simulink model "Project26"  (R2023b)
settings: Solver=ode4  StartTime=0.0  StopTime=4*pi/n  FixedStep=0.1  RelTol=1e-3
values from neighbouring files (symbols this model uses):
  A = [A1; A2; A3; A4; A5; A6; A7; A8; A9; A10; A11; A12; A13; A14]    [Main.m]
  a = (509.4*1000+R_E+529.9*1000+R_E)/2    [Main.m]
  A_ssb = zeros(3,3,6)    [Main.m]
  e = 0.00149    [Main.m]
  epsilon = deg2rad(23.45)    [Main.m]
  F_e = 1358+600+150    (= 2108)    [Main.m]
  FOV = deg2rad(114)    [Main.m]
  G = 6.67*10^-11    (= 6.67e-11)    [Main.m]
  I = [Ix 0 0; 0 Iy 0; 0 0 Iz]    [Main.m]
  i = deg2rad(97.525)    [Main.m]
  I_inv = inv(I)    [Main.m]
  Ix = 0.13    [Main.m]
  Iy = 0.16    [Main.m]
  Iz = 0.18    [Main.m]
  j_B = [0.01, 0.05, 0.01]'    [Main.m]
  Mt = 5.97219e24    (= 5.97219e+24)    [Main.m]
  n = sqrt(G*Mt/a^3)    [Main.m]
  N_B = [n1; n2; n3; n4; n5; n6; n7; n8; n9; n10;n11;n12;n13;n14]    [Main.m]
  n_sun = 2*pi/T_earth    (= 1.99238499086e-07)    [Main.m]
  OM = deg2rad(6.934*180/12)    [Main.m]
  om = deg2rad(287.373)    [Main.m]
  q0 = [0 0 0 1]    [Main.m]
  r_CG = [0.02 0 0]    [Main.m]
  R_sun = astroConstants(2)*1e3    [Main.m]
  rF = [rF1; rF2; rF3; rF4; rF5; rF6; rF7; rF8; rF9; rF10;rF11;rF12;rF13;rF14]    [Main.m]
  theta0 = 0    [Main.m]
  Tsample = 0.1    [Main.m]
  w0 = [w_x0 w_y0 w_z0]    [Main.m]
  w_E = 7.291597763887421e-05    (= 7.29159776389e-05)    [Main.m]
  w_LN = [0 0 n]    [Main.m]
undefined symbols (not defined in the file or in its folder): actuators, control, DiscIntNeverNeededParam, environment, magnitude, sensors, settings
libraries: vrlib x6, matrix_library x5, simulink x2, aerolibutil x1
(part 1 of 2)
settings Model: Creator=aless  LastModifiedBy=aless

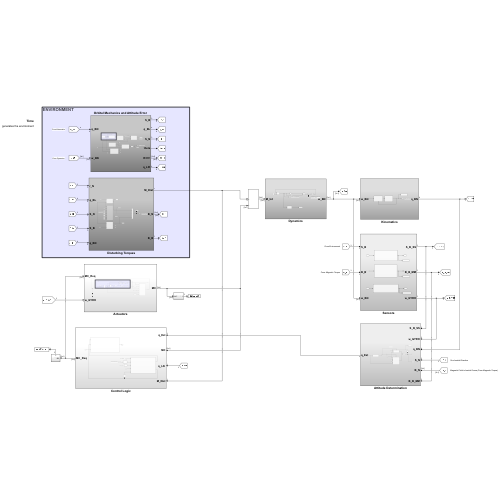
[thumbnail: Simulink's stored preview of the top-level diagram]
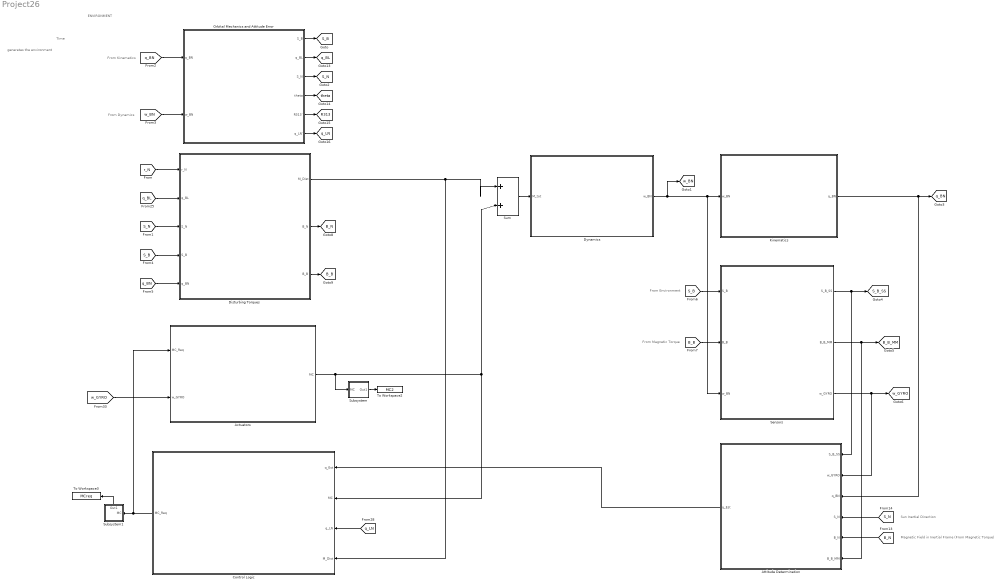
== system Project26 ==
  note: ENVIRONMENT
  note: generates the environment
  note: Time
  note: From Kinematics
  note: From Dynamics
  note: From Magnetic Torque
  note: From Environment
  note: Magnetic Field in Inertial Frame (From Magnetic Torque)
  note: Sun Inertial Direction
  Actuators : Subsystem
  Attitude Determination : Subsystem
  Control Logic : Subsystem
  Disturbing Torques : Subsystem
  Dynamics : Subsystem
  Kinematics : Subsystem
  "Orbital Mechanics and Attitude Error " : Subsystem
  Sensors : Subsystem
  Subsystem : Subsystem
  Subsystem1 : Subsystem
      settings: PortSchema="{\"entries\":[{\"content\":{\"sides\":[{\"content\":{},\"type\":\"ConnectorPlacement.EquallySpacedRectSide\",\"uuid\":\"79d52842-7462-4863-bae2-aaedde0a1e4a\"},{\"content\":{\"connectorIds\":[\"Out1\"],\"side\":\"RIGHT\"},\"type\":\"ConnectorPlacement.EquallySpacedRectSide\",\"uuid\":\"6db4fd27-b070-41dc-87e0-3dbfd9c74019\"},{\"content\":{\"side\":\"TOP\"},\"type\":\"ConnectorPlacement.EquallySpacedRectSide\",\"uuid\":\"0b737283-1eca-4b40-8e8f-9cc579166d68\"},{\"content\":{\"connectorIds\":[\"In1\"],\"side\":\"BOTTOM\"},\"type\":\"ConnectorPlacement.EquallySpacedRectSide\",\"uuid\":\"dd012077-7228-4314-a421-234f34c87179\"}]},\"type\":\"ConnectorPlacement.EquallySpacedConnector\",\"uuid\":\"e026e30a-a92e-42fe-b6eb-86c750f20789\"}],\"packageUris\":[\"http://schema.mathworks.com/mf0/Connector/R2020b\"],\"version\":\"1.0\"}"
  Sum : Sum  Inputs=|++
  To Workspace2 : ToWorkspace  VariableName=MC2  SampleTime=-1
  To Workspace3 : ToWorkspace  VariableName=MCreq  SampleTime=-1
  tag scope: B_B=global, B_B_MM=global, B_N=global, R313=global, S_B=global, S_B_SS=global, S_N=global, q_BL=global, q_BN=global, q_LN=global, theta=global, w_BN=global, w_GYRO=global
  wires:
  [w_BN] -> "Orbital Mechanics and Attitude Error "/2(w_BN)
  [q_BN] -> "Orbital Mechanics and Attitude Error "/1(q_BN)
  "Orbital Mechanics and Attitude Error "/1(S_B) -> [S_B]
  [S_N] -> Disturbing Torques/3(S_N)
  [r_N] -> Disturbing Torques/1(r_N)
  [S_B] -> Disturbing Torques/4(S_B)
  [q_BN] -> Disturbing Torques/5(q_BN)
  "Orbital Mechanics and Attitude Error "/3(S_N) -> [S_N]
  Kinematics/1(q_BN) -> Attitude Determination/3(q_BN), [q_BN]
  [S_B] -> Sensors/1(S_B)
  [B_B] -> Sensors/2(B_B)
  Sensors/1(S_B_SS) -> [S_B_SS], Attitude Determination/1(S_B_SS)
  Sensors/2(B_B_MM) -> [B_B_MM], Attitude Determination/6(B_B_MM)
  Sensors/3(w_GYRO) -> [w_GYRO], Attitude Determination/2(w_GYRO)
  Disturbing Torques/2(B_N) -> [B_N]
  Disturbing Torques/3(B_B) -> [B_B]
  Sum/1 -> Dynamics/1(M_tot)
  "Orbital Mechanics and Attitude Error "/2(q_BL) -> [q_BL]
  [q_BL] -> Disturbing Torques/2(q_BL)
  "Orbital Mechanics and Attitude Error "/4(theta) -> [theta]
  "Orbital Mechanics and Attitude Error "/5(R313') -> [R313]
  "Orbital Mechanics and Attitude Error "/6(q_LN') -> [q_LN]
  [w_GYRO] -> Actuators/1(w_GYRO)
  Actuators/1(MC) -> Sum/2, Control Logic/2(MC), Subsystem/1(MC)
  Subsystem/1(Out1) -> To Workspace2/1
  Subsystem1/1(Out1) -> To Workspace3/1
  Disturbing Torques/1(M_Dist) -> Control Logic/4(M_Dist), Sum/1
  Dynamics/1(w_BN) -> [w_BN], Sensors/3(w_BN), Kinematics/1(w_BN)
  [B_N] -> Attitude Determination/5(B_N)
  [S_N] -> Attitude Determination/4(S_N)
  Attitude Determination/1(q_Est) -> Control Logic/1(q_Est)
  [q_LN] -> Control Logic/3("q_LN ")
  Control Logic/1(MC_Req) -> Subsystem1/1(MC), Actuators/2(MC_Req)

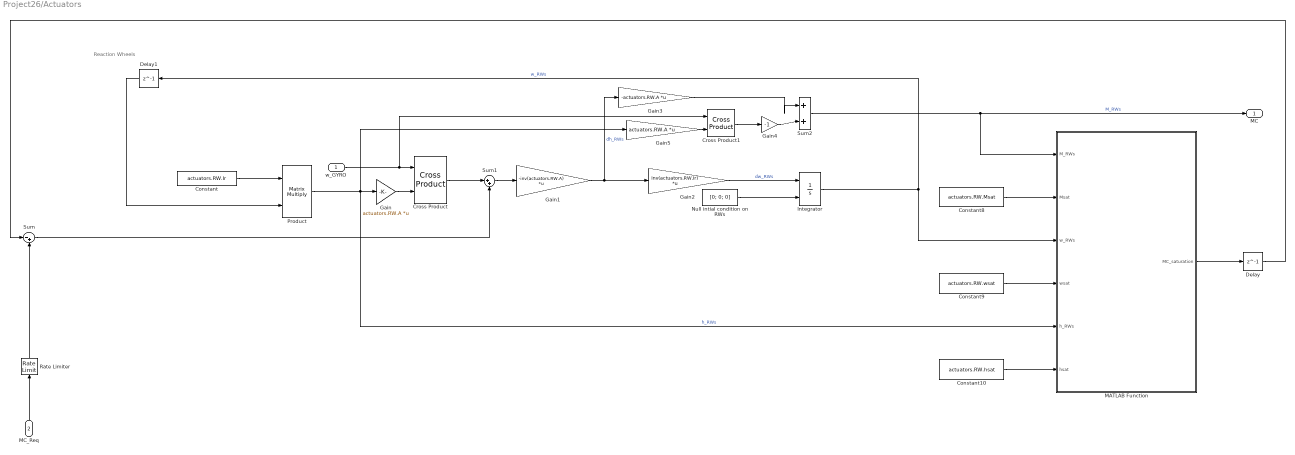
== system Project26/Actuators ==
  note: Reaction Wheels
  w_GYRO : Inport
  MC_Req : Inport  Port=2
  Constant : Constant  Value=actuators.RW.Ir
  Constant10 : Constant  Value=actuators.RW.hsat
  Constant8 : Constant  Value=actuators.RW.Msat
  Constant9 : Constant  Value=actuators.RW.wsat
  Cross Product : matrix_library/Cross Product
  Cross Product1 : matrix_library/Cross Product
  Delay : Delay  DelayLength=1
  Delay1 : Delay  DelayLength=1  InitialCondition=0
  Gain : Gain  Gain=actuators.RW.A  Multiplication=Matrix(K*u)
  Gain1 : Gain  Gain=-inv(actuators.RW.A)  Multiplication=Matrix(K*u)
  Gain2 : Gain  Gain=inv(actuators.RW.Ir)  Multiplication=Matrix(K*u)
  Gain3 : Gain  Gain=-actuators.RW.A  Multiplication=Matrix(K*u)
  Gain4 : Gain  Gain=-1
  Gain5 : Gain  Gain=actuators.RW.A  Multiplication=Matrix(K*u)
  Integrator : Integrator  InitialConditionSource=external
  MATLAB Function : MATLAB Function  TreatAsAtomicUnit=on
  Null intial condition on RWs : Constant  Value=[0; 0; 0]
  Product : Product  Multiplication=Matrix(*)
  Rate Limiter : RateLimiter
  Sum : Sum  Inputs=|-+
  Sum1 : Sum  Inputs=|++
  Sum2 : Sum  Inputs=|++
  MC : Outport
  wires:
  Sum/1 -> Sum1/2
  Sum2/1 -> MC/1, MATLAB Function/1(M_RWs)  "M_RWs"
  Gain2/1 -> Integrator/1  "dw_RWs"
  Gain3/1 -> Sum2/1
  Gain/1 -> Cross Product/2
  Delay1/1 -> Product/2
  w_GYRO/1 -> Cross Product1/1, Cross Product/1
  Gain1/1 -> Gain2/1, Gain3/1  "dh_RWs"
  Constant/1 -> Product/1
  Constant10/1 -> MATLAB Function/6(hsat)
  Delay/1 -> Sum/1
  MATLAB Function/1(MC_saturation) -> Delay/1
  Integrator/1 -> MATLAB Function/3(w_RWs), Delay1/1  "w_RWs"
  Product/1 -> MATLAB Function/5(h_RWs), Gain/1, Gain5/1  "h_RWs"
  Sum1/1 -> Gain1/1
  Gain5/1 -> Cross Product1/2
  Constant8/1 -> MATLAB Function/2(Msat)
  Constant9/1 -> MATLAB Function/4(wsat)
  Cross Product1/1 -> Gain4/1
  Cross Product/1 -> Sum1/1
  Gain4/1 -> Sum2/2
  Null intial condition on RWs/1 -> Integrator/2
  MC_Req/1 -> Rate Limiter/1
  Rate Limiter/1 -> Sum/2

== system Project26/Attitude Determination ==
  note: YES (isNaN = true)
  S_B_SS : Inport
  w_GYRO : Inport  Port=2
  q_BN : Inport  Port=3
  S_N : Inport  Port=4
  B_N : Inport  Port=5
  B_B_MM : Inport  Port=6
  Delay : Delay  DelayLength=1
  Enabled Subsystem : Subsystem  TreatAsAtomicUnit=on
  Enabled Subsystem1 : Subsystem  TreatAsAtomicUnit=on
  Merge1 : Merge
  NOT (Change of condition) : Logic  Operator=NOT  IconShape=distinctive  AllPortsSameDT=off  OutDataTypeStr=boolean
  Out of FOV check : Subsystem
  To Workspace : ToWorkspace  VariableName=delay  SaveFormat=Timeseries  SampleTime=-1
  To Workspace9 : ToWorkspace  VariableName=q_Est  SampleTime=-1
  q_Est : Outport
  wires:
  S_B_SS/1 -> Enabled Subsystem1/5(S_B_SS), Out of FOV check/1(S_B_SS)
  Out of FOV check/1(Out1) -> NOT (Change of condition)/1, Enabled Subsystem/Enable
  w_GYRO/1 -> Enabled Subsystem/1(w_GYRO)
  q_BN/1 -> Enabled Subsystem1/1(q_BN), Enabled Subsystem/3(q_BN)
  Enabled Subsystem/1(q_est) -> Merge1/1
  Merge1/1 -> To Workspace9/1, q_Est/1, Delay/1
  Delay/1 -> To Workspace/1, Enabled Subsystem/2(q_0)
  Enabled Subsystem1/1(q_est) -> Merge1/2
  NOT (Change of condition)/1 -> Enabled Subsystem1/Enable
  S_N/1 -> Enabled Subsystem1/2(S_N)
  B_N/1 -> Enabled Subsystem1/3(B_N)
  B_B_MM/1 -> Enabled Subsystem1/4(B_B_MM)

== system Project26/Control Logic ==
  note: From Actuators
  note: From Attitude Determination
  note: From Gyroscopes
  q_Est : Inport
  MC : Inport  Port=2
  "q_LN " : Inport  Port=3
  M_Dist : Inport  Port=4
  Control Block : Subsystem
  Delay : Delay  DelayLength=1
  Normalize Vector2 : vrlib/Utilities/Normalize Vector  maxzero=0
  State Observer : Subsystem
  MC_Req : Outport
  wires:
  q_Est/1 -> Normalize Vector2/1
  [w_GYRO] -> State Observer/3(w_GYRO)
  Delay/1 -> State Observer/5(q_obs_delay)
  Normalize Vector2/1 -> State Observer/2(q_raw)
  Control Block/1(MC_Req) -> MC_Req/1
  State Observer/2(q_obs) -> Control Block/2(q_obs), Delay/1
  State Observer/1(w_obs) -> Control Block/1(w_obs)
  MC/1 -> State Observer/1(MC_est)
  "q_LN "/1 -> Control Block/3("q_LN ")
  M_Dist/1 -> State Observer/4(MD)

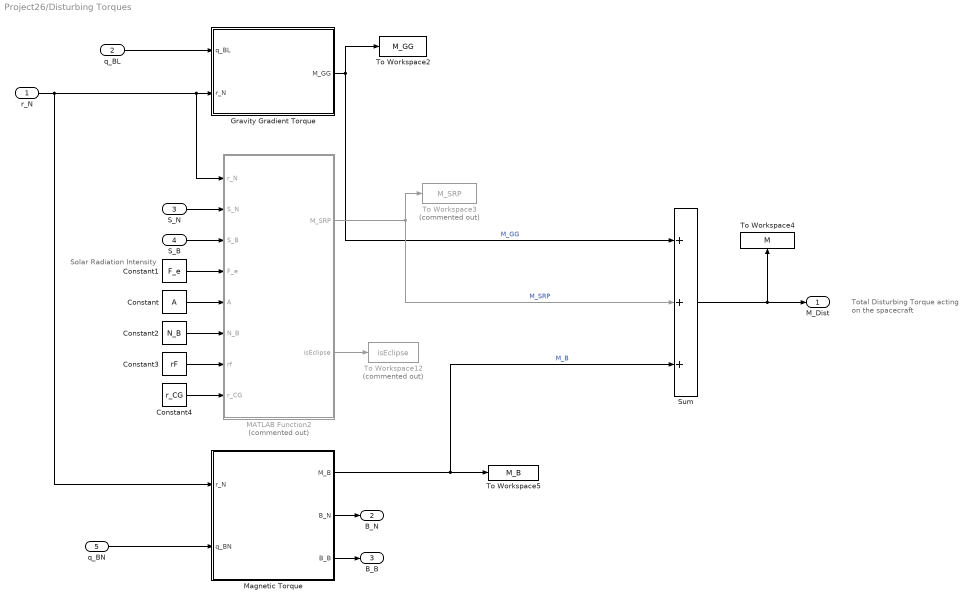
== system Project26/Disturbing Torques ==
  note: Total Disturbing Torque
      | acting on the spacecraft
  note: Solar Radiation Intensity
  r_N : Inport
  q_BL : Inport  Port=2
  S_N : Inport  Port=3
  S_B : Inport  Port=4
  q_BN : Inport  Port=5
  Constant : Constant  Value=A
  Constant1 : Constant  Value=F_e
  Constant2 : Constant  Value=N_B
  Constant3 : Constant  Value=rF
  Constant4 : Constant  Value=r_CG
  Gravity Gradient Torque : Subsystem
  MATLAB Function2 : MATLAB Function  Commented=on  TreatAsAtomicUnit=on
  Magnetic Torque : Subsystem
  Sum : Sum  Inputs=+++
  To Workspace12 : ToWorkspace  Commented=on  VariableName=isEclipse  SampleTime=-1
  To Workspace2 : ToWorkspace  VariableName=M_GG  SampleTime=-1
  To Workspace3 : ToWorkspace  Commented=on  VariableName=M_SRP  SampleTime=-1
  To Workspace4 : ToWorkspace  VariableName=M  SampleTime=-1
  To Workspace5 : ToWorkspace  VariableName=M_B  SampleTime=-1
  M_Dist : Outport
  B_N : Outport  Port=2
  B_B : Outport  Port=3
  wires:
  Constant1/1 -> MATLAB Function2/4(F_e)
  q_BL/1 -> Gravity Gradient Torque/1(q_BL)
  r_N/1 -> MATLAB Function2/1(r_N), Gravity Gradient Torque/2(r_N), Magnetic Torque/1(r_N)
  MATLAB Function2/2(isEclipse) -> To Workspace12/1
  q_BN/1 -> Magnetic Torque/2(q_BN)
  Sum/1 -> M_Dist/1, To Workspace4/1
  Gravity Gradient Torque/1(M_GG) -> To Workspace2/1, Sum/1  "M_GG"
  Magnetic Torque/1(M_B) -> Sum/3, To Workspace5/1  "M_B"
  S_N/1 -> MATLAB Function2/2(S_N)
  S_B/1 -> MATLAB Function2/3(S_B)
  Magnetic Torque/2(B_N) -> B_N/1
  Magnetic Torque/3(B_B) -> B_B/1
  Constant/1 -> MATLAB Function2/5(A)
  Constant2/1 -> MATLAB Function2/6(N_B)
  MATLAB Function2/1(M_SRP) -> To Workspace3/1, Sum/2  "M_SRP"
  Constant3/1 -> MATLAB Function2/7(rf)
  Constant4/1 -> MATLAB Function2/8(r_CG)

== system Project26/Dynamics ==
  note: Total Disturbing Torque+Control
      | acting on the spacecraft
  note: Angular velocity ( Body Frame )
  note: w
  M_tot : Inport
  Cross Product : vrlib/Utilities/Cross Product
  Gain : Gain  Gain=I  Multiplication=Matrix(K*u)
  Gain1 : Gain  Gain=I_inv  Multiplication=Matrix(K*u)
  Initial Condition : Constant  Value=w0
  Integrator : Integrator  InitialConditionSource=external
  Subsystem : Subsystem
  Sum : Sum  Inputs=|++
  To Workspace1 : ToWorkspace  VariableName=omega  SampleTime=-1
  w_BN : Outport
  wires:
  M_tot/1 -> Sum/2
  Gain1/1 -> Integrator/1
  Initial Condition/1 -> Integrator/2
  Sum/1 -> Gain1/1
  Gain/1 -> Cross Product/1  "I*w"
  Cross Product/1 -> Sum/1
  Integrator/1 -> Subsystem/1(MC), w_BN/1, Cross Product/2, Gain/1
  Subsystem/1(Out1) -> To Workspace1/1

== system Project26/Kinematics ==
  note: (Body Frame Quaternion)
  w_BN : Inport
  Quaternion Normalisation : Subsystem
  Quaternions : Subsystem
      settings: PortSchema="{\"entries\":[{\"content\":{\"sides\":[{\"content\":{\"connectorIds\":[\"In1\"]},\"type\":\"ConnectorPlacement.EquallySpacedRectSide\",\"uuid\":\"337480c7-b996-434a-97d1-93b75d8b293c\"},{\"content\":{\"connectorIds\":[\"Out1\"],\"side\":\"RIGHT\"},\"type\":\"ConnectorPlacement.EquallySpacedRectSide\",\"uuid\":\"41d32615-4344-48a4-ad5b-2dad4deabdda\"},{\"content\":{\"side\":\"TOP\"},\"type\":\"ConnectorPlacement.EquallySpacedRectSide\",\"uuid\":\"47835596-097d-48d1-90ae-77b48fddf76d\"},{\"content\":{\"connectorIds\":[\"In2\"],\"side\":\"BOTTOM\"},\"type\":\"ConnectorPlacement.EquallySpacedRectSide\",\"uuid\":\"9f38fa4d-c6c1-4321-9750-02b4f73c744f\"}]},\"type\":\"ConnectorPlacement.EquallySpacedConnector\",\"uuid\":\"8ea16f6d-57f4-43cd-ae9c-44a64026dd8f\"}],\"packageUris\":[\"http://schema.mathworks.com/mf0/Connector/R2020b\"],\"version\":\"1.0\"}"
  To Workspace : ToWorkspace  VariableName=q_BN  SampleTime=-1
  q_BN : Outport
  wires:
  w_BN/1 -> Quaternions/1(w)
  Quaternion Normalisation/1(q_BN) -> To Workspace/1, q_BN/1, Quaternions/2(q_BN)
  Quaternions/1(q(t)) -> Quaternion Normalisation/1(q(t))

== system Project26/Orbital Mechanics and Attitude Error  ==
  note: r_N = r ( Inertial Frame )
  note: Sun Direction ( Body Frame )
  note: r ( Body Frame )
  note: Two-Body Keplerian Dynamics
  q_BN : Inport
  w_BN : Inport  Port=2
  " Rotation from Inertial to Body Frame" : Subsystem
  Attitude Error : Subsystem
  Computation of r (vector) : Subsystem
  Normalize Vector : vrlib/Utilities/Normalize Vector  maxzero=0
  Rotation from Inertial to Body Frame : Subsystem
  Sun Inertial Direction : Subsystem
  Theta angle : Subsystem
  To Workspace : ToWorkspace  VariableName=r_B  SampleTime=-1
  To Workspace1 : ToWorkspace  VariableName=S_B  SampleTime=-1
  r (Magnitude) : Subsystem
  S_B : Outport
  q_BL : Outport  Port=2
  S_N : Outport  Port=3
  theta : Outport  Port=4
  R313' : Outport  Port=5
  q_LN' : Outport  Port=6
  wires:
  Theta angle/1(theta) -> Attitude Error/1(Theta), theta/1, Computation of r (vector)/2(theta), r (Magnitude)/1(theta)
  r (Magnitude)/1("r ") -> Computation of r (vector)/1(r)
  Computation of r (vector)/1(r_N) -> " Rotation from Inertial to Body Frame"/1(r_N)
  Sun Inertial Direction/1(S_N) -> Rotation from Inertial to Body Frame/1(S_N), S_N/1
  " Rotation from Inertial to Body Frame"/1(r_B) -> To Workspace/1
  Rotation from Inertial to Body Frame/1(S_B) -> Normalize Vector/1
  Normalize Vector/1 -> S_B/1, To Workspace1/1
  Attitude Error/1(q_BL) -> q_BL/1
  w_BN/1 -> Attitude Error/3(w_BN)
  q_BN/1 -> " Rotation from Inertial to Body Frame"/2(q_BN), Attitude Error/2(q_BN), Rotation from Inertial to Body Frame/2(q_BN)
  Computation of r (vector)/2(R313') -> R313'/1
  Attitude Error/2(q_LN') -> q_LN'/1

== system Project26/Sensors ==
  S_B : Inport
  B_B : Inport  Port=2
  w_BN : Inport  Port=3
  Gyroscopes : Subsystem
  Magnetometer : Subsystem
  Sun Sensor : Subsystem
      settings: PortSchema="{\"entries\":[{\"content\":{\"sides\":[{\"content\":{},\"type\":\"ConnectorPlacement.EquallySpacedRectSide\",\"uuid\":\"8c40b47c-c81f-4db9-9ecd-3bac70546829\"},{\"content\":{\"side\":\"RIGHT\"},\"type\":\"ConnectorPlacement.EquallySpacedRectSide\",\"uuid\":\"47b5da33-6a3e-4432-914f-62c5c8f09690\"},{\"content\":{\"connectorIds\":[\"In1\"],\"side\":\"TOP\"},\"type\":\"ConnectorPlacement.EquallySpacedRectSide\",\"uuid\":\"b24e362e-8249-41df-bcdf-30c7d216309c\"},{\"content\":{\"connectorIds\":[\"Out1\"],\"side\":\"BOTTOM\"},\"type\":\"ConnectorPlacement.EquallySpacedRectSide\",\"uuid\":\"ca1f88ba-b9cd-4169-975e-ff1bd0c05719\"}]},\"type\":\"ConnectorPlacement.EquallySpacedConnector\",\"uuid\":\"37a9beb8-71a0-43e5-b724-5b60e3432ba4\"}],\"packageUris\":[\"http://schema.mathworks.com/mf0/Connector/R2020b\"],\"version\":\"1.0\"}"
  To Workspace : ToWorkspace  VariableName=w_measured  SampleTime=-1
  To Workspace1 : ToWorkspace  VariableName=S_B_meas  SampleTime=-1
  To Workspace2 : ToWorkspace  VariableName=B_B_meas  SampleTime=-1
  S_B_SS : Outport
  B_B_MM : Outport  Port=2
  w_GYRO : Outport  Port=3
  wires:
  S_B/1 -> Sun Sensor/1(S_B)
  w_BN/1 -> Gyroscopes/1(w_BN)
  Sun Sensor/1(S_B_SS) -> S_B_SS/1, To Workspace1/1
  Magnetometer/1(B_B_MM) -> B_B_MM/1, To Workspace2/1
  Gyroscopes/1(w_GYRO) -> w_GYRO/1, To Workspace/1
  B_B/1 -> Magnetometer/1(B_B)

== system Project26/Subsystem ==
  MC : Inport
  Demux : Demux  Outputs=3
  Mux : Mux  Inputs=3
  Out1 : Outport
  wires:
  MC/1 -> Demux/1
  Demux/1 -> Mux/1
  Demux/2 -> Mux/2
  Demux/3 -> Mux/3
  Mux/1 -> Out1/1

== system Project26/Subsystem1 ==
  MC : Inport
  Demux : Demux  Outputs=3
  Mux : Mux  Inputs=3
  Out1 : Outport
  wires:
  MC/1 -> Demux/1
  Demux/1 -> Mux/1
  Demux/2 -> Mux/2
  Demux/3 -> Mux/3
  Mux/1 -> Out1/1

== system Project26/Attitude Determination/Enabled Subsystem ==
  note: Estimated
      | Quaternion
  w_GYRO : Inport
  q_0 : Inport  Port=2
  q_BN : Inport  Port=3
  Enable : EnablePort  StatesWhenEnabling=reset
  Kinematics : Subsystem
  Sign Determination : Subsystem
  To Workspace : ToWorkspace  VariableName=q_estG1  SampleTime=-1
  q_est : Outport
  wires:
  q_BN/1 -> Sign Determination/2(q_BN)
  w_GYRO/1 -> Kinematics/1(w)
  Kinematics/1(q_est) -> Sign Determination/1("q_est "), To Workspace/1
  q_0/1 -> Kinematics/2(q_0)
  Sign Determination/1(q_est) -> q_est/1

== system Project26/Attitude Determination/Enabled Subsystem1 ==
  note: S_B_Estim
  q_BN : Inport
  S_N : Inport  Port=2
  B_N : Inport  Port=3
  B_B_MM : Inport  Port=4
  S_B_SS : Inport  Port=5
  Enable : EnablePort
  Attitude determination : MATLAB Function  TreatAsAtomicUnit=on
  Constant : Constant  Value=sensors.mag.accuracy
  Constant2 : Constant  Value=sensors.SS.accuracy
  Normalize Vector1 : vrlib/Utilities/Normalize Vector  maxzero=0
  Sign determination : Subsystem
  q_est : Outport
  wires:
  Constant/1 -> Attitude determination/1(a_mag)
  q_BN/1 -> Sign determination/2(q_BN)
  Constant2/1 -> Attitude determination/2(a_sun)
  Normalize Vector1/1 -> Attitude determination/3(S_N)
  S_B_SS/1 -> Attitude determination/4(S_B_Estim)
  S_N/1 -> Normalize Vector1/1
  B_N/1 -> Attitude determination/5(B_N)
  B_B_MM/1 -> Attitude determination/6(B_B_Estim)
  Sign determination/1(q_0) -> q_est/1
  Attitude determination/1(q_est) -> Sign determination/1("q_est ")

== system Project26/Attitude Determination/Out of FOV check ==
  note: If at least one component is NaN, the Sun is not in the FOV
  S_B_SS : Inport
  Demux : Demux  Outputs=3
  IsNaN : RelationalOperator  Operator=isNaN  OutDataTypeStr=boolean  RndMeth=Simplest  InputSameDT=off
  Out1 : Outport
  wires:
  S_B_SS/1 -> Demux/1
  Demux/1 -> IsNaN/1
  IsNaN/1 -> Out1/1

== system Project26/Control Logic/Control Block ==
  note: Global Pointing Error
  note: Control Algorithms
  note: Mission Phase Decision
  w_obs : Inport
  q_obs : Inport  Port=2
  "q_LN " : Inport  Port=3
  Clock : Clock
  Constant : Constant  Value=control.detumbling.MaxTime
  Constant1 : Constant  Value=control.slewManeuvre.MaxTime
  Detumbling : Subsystem  TreatAsAtomicUnit=on
  If : If  NumInputs=3  IfExpression=u1<=u2  ElseIfExpressions=u2<u1<=u3
  Merge : Merge  Inputs=3
  Merge1 : Merge  Inputs=3
  Slew Maneuvre : Subsystem  TreatAsAtomicUnit=on
  To Workspace : ToWorkspace  VariableName=pointing_err  SampleTime=-1
  Trajectory Tracking : Subsystem  TreatAsAtomicUnit=on
  MC_Req : Outport
  wires:
  Constant1/1 -> If/3
  Constant/1 -> If/2
  Clock/1 -> If/1
  If/1 -> Detumbling/Action
  If/2 -> Slew Maneuvre/Action
  If/3 -> Trajectory Tracking/Action
  q_obs/1 -> Detumbling/2(q_obs), Trajectory Tracking/2(q_obs), Slew Maneuvre/2(q_obs)
  w_obs/1 -> Detumbling/1(w_obs), Trajectory Tracking/1(w_obs), Slew Maneuvre/1(w_obs)
  Trajectory Tracking/2(Pointing Error) -> Merge/1
  Slew Maneuvre/2(Pointing Error (SM)) -> Merge/2
  Detumbling/2(Pointing Error (DT)) -> Merge/3
  Merge/1 -> To Workspace/1
  Slew Maneuvre/1(MC) -> Merge1/2
  Trajectory Tracking/1(MC) -> Merge1/3
  Merge1/1 -> MC_Req/1  "MC_required"
  Detumbling/1(MC) -> Merge1/1
  "q_LN "/1 -> Detumbling/3(q_LN), Slew Maneuvre/3(q_LN), Trajectory Tracking/3(q_LN)

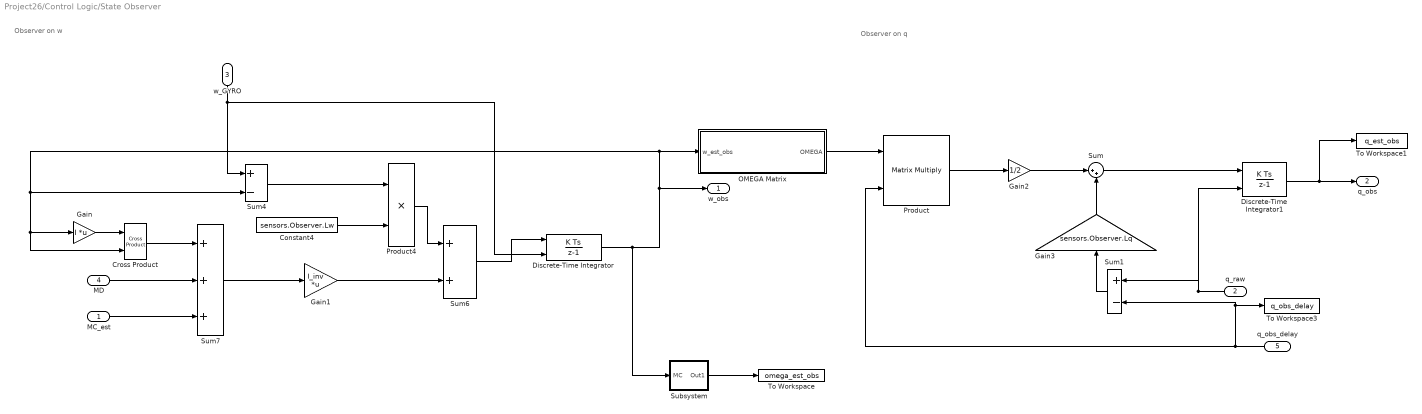
== system Project26/Control Logic/State Observer ==
  note: Observer on q
  note: Observer on w
  MC_est : Inport
  q_raw : Inport  Port=2
  w_GYRO : Inport  Port=3
  MD : Inport  Port=4
  q_obs_delay : Inport  Port=5
  Constant4 : Constant  Value=sensors.Observer.Lw
  Cross Product : vrlib/Utilities/Cross Product
  Discrete-Time Integrator : DiscreteIntegrator  InitialConditionSource=external  InitialCondition=sensors.Observer.w0  SampleTime=Tsample  ICPrevOutput=DiscIntNeverNeededParam  ICPrevScaledInput=DiscIntNeverNeededParam
  Discrete-Time Integrator1 : DiscreteIntegrator  InitialConditionSource=external  SampleTime=Tsample  ICPrevOutput=DiscIntNeverNeededParam  ICPrevScaledInput=DiscIntNeverNeededParam
  Gain : Gain  Gain=I  Multiplication=Matrix(K*u)
  Gain1 : Gain  Gain=I_inv  Multiplication=Matrix(K*u)
  Gain2 : Gain  Gain=1/2
  Gain3 : Gain  Gain=sensors.Observer.Lq
  OMEGA Matrix : Subsystem
  Product : Product  Multiplication=Matrix(*)
  Product4 : Product
  Subsystem : Subsystem
  Sum : Sum  Inputs=|++
  Sum1 : Sum  Inputs=|+-
  Sum4 : Sum  Inputs=+-
  Sum6 : Sum
  Sum7 : Sum  Inputs=+++
  To Workspace : ToWorkspace  VariableName=omega_est_obs  SampleTime=-1
  To Workspace1 : ToWorkspace  VariableName=q_est_obs  SampleTime=-1
  To Workspace3 : ToWorkspace  VariableName=q_obs_delay  SampleTime=-1
  w_obs : Outport
  q_obs : Outport  Port=2
  wires:
  Product4/1 -> Sum6/1
  Cross Product/1 -> Sum7/1
  Gain1/1 -> Sum6/2
  MC_est/1 -> Sum7/3
  Discrete-Time Integrator/1 -> Subsystem/1(MC), w_obs/1, Sum4/2, Gain/1, Cross Product/2, OMEGA Matrix/1(w_est_obs)
  Sum4/1 -> Product4/1
  Gain/1 -> Cross Product/1
  Constant4/1 -> Product4/2
  Sum7/1 -> Gain1/1
  w_GYRO/1 -> Discrete-Time Integrator/2, Sum4/1
  OMEGA Matrix/1(OMEGA) -> Product/1
  Product/1 -> Gain2/1
  Gain2/1 -> Sum/1
  Gain3/1 -> Sum/2
  Sum1/1 -> Gain3/1
  q_obs_delay/1 -> Sum1/2, To Workspace3/1, Product/2
  Sum/1 -> Discrete-Time Integrator1/1
  Sum6/1 -> Discrete-Time Integrator/1
  MD/1 -> Sum7/2
  Discrete-Time Integrator1/1 -> q_obs/1, To Workspace1/1
  q_raw/1 -> Discrete-Time Integrator1/2, Sum1/1
  Subsystem/1(Out1) -> To Workspace/1

== system Project26/Disturbing Torques/Gravity Gradient Torque ==
  note: Torque due to
      | Gravity Gradient
  note: c1c3
  note: c2c3
  note: c2c1
  note: c1,c2,c3
  q_BL : Inport
  r_N : Inport  Port=2
  Constant1 : Constant  Value=3
  Cubic Power : Math  Operator=pow
  Demux : Demux  Outputs=3
  Divide : Product  Inputs=*/
  Gain : Gain  Gain=(Iz-Iy)
  Gain1 : Gain  Gain=(Ix-Iz)
  Gain2 : Gain  Gain=(Iy-Ix)
  Gain7 : Gain  Gain=3*G*Mt
  Mux : Mux  Inputs=3
  Normalisation : Subsystem
  Product : Product
  Product1 : Product
  Product2 : Product
  Rotation of vector [1 0 0] : Subsystem
  Vector : Constant  Value=[1 0 0]'
  M_GG : Outport
  wires:
  Cubic Power/1 -> Divide/2
  Demux/1 -> Product1/1, Product2/2
  q_BL/1 -> Rotation of vector [1 0 0]/1(q_BL)
  Rotation of vector [1 0 0]/1(v_rot) -> Demux/1
  Normalisation/1(R) -> Cubic Power/1
  Divide/1 -> M_GG/1
  Vector/1 -> Rotation of vector [1 0 0]/2(Vector [1 0 0])  "vect"
  Product2/1 -> Gain2/1
  Demux/2 -> Product/1, Product2/1
  Mux/1 -> Gain7/1
  r_N/1 -> Normalisation/1(r_N)
  Gain7/1 -> Divide/1
  Demux/3 -> Product1/2, Product/2
  Constant1/1 -> Cubic Power/2
  Gain/1 -> Mux/1
  Gain1/1 -> Mux/2
  Gain2/1 -> Mux/3
  Product1/1 -> Gain1/1
  Product/1 -> Gain/1

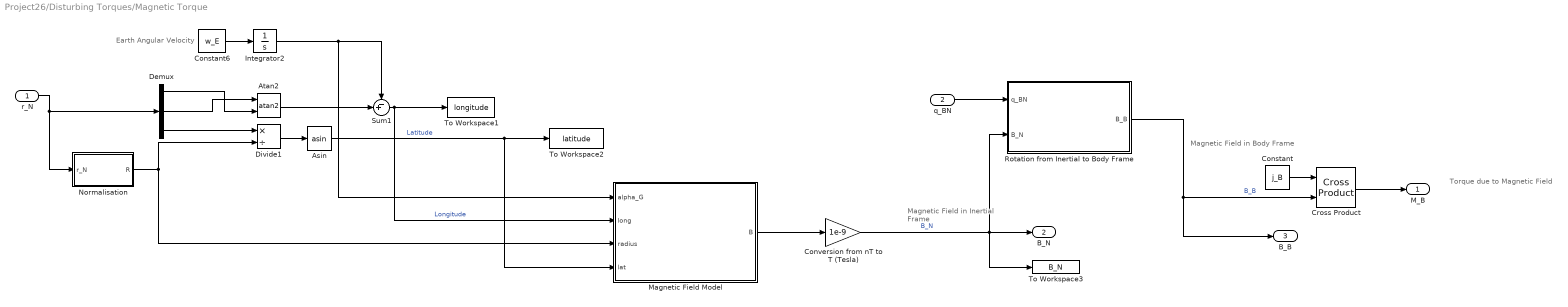
== system Project26/Disturbing Torques/Magnetic Torque ==
  note: Magnetic Field
      | in Body Frame
  note: Magnetic Field
      | in Inertial Frame
  note: Earth Angular Velocity
  note: Torque due to
      | Magnetic Field
  r_N : Inport
  q_BN : Inport  Port=2
  Asin : Trigonometry  Operator=asin
  Atan2 : Trigonometry  Operator=atan2
  Constant : Constant  Value=j_B
  Constant6 : Constant  Value=w_E
  Conversion from nT to T (Tesla) : Gain  Gain=1e-9
  Cross Product : matrix_library/Cross Product
  Demux : Demux  Outputs=3
  Divide1 : Product  Inputs=*/
  Integrator2 : Integrator
  Magnetic Field Model : MATLAB Function  TreatAsAtomicUnit=on
  Normalisation : Subsystem
  Rotation from Inertial to Body Frame : Subsystem
  Sum1 : Sum  Inputs=-+|
  To Workspace1 : ToWorkspace  VariableName=longitude  SampleTime=-1
  To Workspace2 : ToWorkspace  VariableName=latitude  SampleTime=-1
  To Workspace3 : ToWorkspace  VariableName=B_N  SampleTime=-1
  M_B : Outport
  B_N : Outport  Port=2
  B_B : Outport  Port=3
  wires:
  Demux/2 -> Atan2/1
  Demux/3 -> Divide1/1
  Atan2/1 -> Sum1/2
  Normalisation/1(R) -> Magnetic Field Model/3(radius), Divide1/2
  Demux/1 -> Atan2/2
  Divide1/1 -> Asin/1
  Asin/1 -> Magnetic Field Model/4(lat), To Workspace2/1  "Latitude"
  Constant6/1 -> Integrator2/1
  Sum1/1 -> To Workspace1/1, Magnetic Field Model/2(long)  "Longitude"
  r_N/1 -> Normalisation/1(r_N), Demux/1
  Integrator2/1 -> Sum1/1, Magnetic Field Model/1(alpha_G)
  Rotation from Inertial to Body Frame/1(B_B) -> B_B/1, Cross Product/2  "B_B"
  Constant/1 -> Cross Product/1
  Magnetic Field Model/1(B) -> Conversion from nT to T (Tesla)/1
  q_BN/1 -> Rotation from Inertial to Body Frame/1(q_BN)
  Cross Product/1 -> M_B/1
  Conversion from nT to T (Tesla)/1 -> B_N/1, Rotation from Inertial to Body Frame/2(B_N), To Workspace3/1  "B_N"

== system Project26/Dynamics/Subsystem ==
  MC : Inport
  Demux : Demux  Outputs=3
  Mux : Mux  Inputs=3
  Out1 : Outport
  wires:
  MC/1 -> Demux/1
  Demux/1 -> Mux/1
  Demux/2 -> Mux/2
  Demux/3 -> Mux/3
  Mux/1 -> Out1/1

== system Project26/Kinematics/Quaternion Normalisation ==
  q(t) : Inport
  Divide : Product  Inputs=*/
  Dot Product : DotProduct  OutDataTypeStr=Inherit: Inherit via internal rule
  Sqrt : Sqrt
  q_BN : Outport
  wires:
  Dot Product/1 -> Sqrt/1
  q(t)/1 -> Divide/1, Dot Product/1, Dot Product/2
  Sqrt/1 -> Divide/2
  Divide/1 -> q_BN/1

== system Project26/Kinematics/Quaternions ==
  note: Normalised
      | quaternion
  w : Inport
  q_BN : Inport  Port=2
  Gain : Gain  Gain=1/2
  Initial Condition : Constant  Value=q0
  Integrator : Integrator  InitialConditionSource=external
  Matrix Multiply : Product  Multiplication=Matrix(*)
  OMEGA Matrix : Subsystem
  q(t) : Outport
  wires:
  Integrator/1 -> q(t)/1
  Initial Condition/1 -> Integrator/2
  Matrix Multiply/1 -> Integrator/1
  Gain/1 -> Matrix Multiply/1
  w/1 -> OMEGA Matrix/1(w)
  OMEGA Matrix/1(OM Matrix) -> Gain/1
  q_BN/1 -> Matrix Multiply/2

== system Project26/Orbital Mechanics and Attitude Error / Rotation from Inertial to Body Frame ==
  note: Quaternion Rotation (Double Tensor Product)
  note: $\vec{r_B} = q_{BN}'\otimes [\vec{r_N};0]\otimes q_{BN}$
  r_N : Inport
  q_BN : Inport  Port=2
  Demux : Demux
  Mux : Mux  Inputs=3
  Quaternion multiplication 1 : Subsystem
  Quaternion multiplication 2 : Subsystem
  Transformation in Quaternion : Subsystem
  Transpose : Gain  Gain=[-1 -1 -1 1]
  r_B : Outport
  wires:
  r_N/1 -> Transformation in Quaternion/1(r_N)
  Mux/1 -> r_B/1
  Transpose/1 -> Quaternion multiplication 1/1(q_BN')
  q_BN/1 -> Quaternion multiplication 2/2(q_BN), Transpose/1
  Transformation in Quaternion/1(q(r_N)) -> Quaternion multiplication 1/2("q(r_N) ")
  Quaternion multiplication 2/1(q(r_B)) -> Demux/1
  Quaternion multiplication 1/1(q1) -> Quaternion multiplication 2/1(q1)
  Demux/1 -> Mux/1
  Demux/2 -> Mux/2
  Demux/3 -> Mux/3

== system Project26/Orbital Mechanics and Attitude Error /Attitude Error ==
  note: Angular Velocity Error
  note: Reference moving attitude
      | (Angular Velocity)
  note: Attitude Error
  note: Reference moving attitude
      | (Quaternion)
  Theta : Inport
  q_BN : Inport  Port=2
  w_BN : Inport  Port=3
  Computation of q_BL : Subsystem
  Constant2 : Constant  Value=w_LN
  Rotation of w_LN : Subsystem
  Sum : Sum  Inputs=|-+
  To Workspace3 : ToWorkspace  VariableName=w_BL  SampleTime=-1
  To Workspace4 : ToWorkspace  VariableName=q_BL  SampleTime=-1
  q_LN : Subsystem
  q_BL : Outport
  q_LN' : Outport  Port=2
  wires:
  Computation of q_BL/1(q_BL) -> Rotation of w_LN/1(q_BL), To Workspace4/1, q_BL/1
  Theta/1 -> q_LN/1(Theta)
  Sum/1 -> To Workspace3/1
  Rotation of w_LN/1(w_LN') -> Sum/1
  Constant2/1 -> Rotation of w_LN/2(w_LN)
  q_BN/1 -> q_LN/2(q_BN), Computation of q_BL/1(q_BN)
  q_LN/1(q_LN') -> Computation of q_BL/2(q_LN'), q_LN'/1
  w_BN/1 -> Sum/2

== system Project26/Orbital Mechanics and Attitude Error /Computation of r (vector) ==
  note: Perifocal Frame
  note: r (Perifocal Frame)
  r : Inport
  theta : Inport  Port=2
  Constant : Constant  Value=0
  Cos1 : Trigonometry  Operator=cos
  Mux1 : Mux  Inputs=3
  Product1 : Product  Multiplication=Matrix(*)
  Product2 : Product
  Rotation (R313') from Perifocal to ECI : Subsystem
  Sin1 : Trigonometry
  To Workspace1 : ToWorkspace  VariableName=r_N  SampleTime=-1
  r_N : Outport
  R313' : Outport  Port=2
  tag scope: r_N=global
  wires:
  Mux1/1 -> Product2/2
  Sin1/1 -> Mux1/2
  Constant/1 -> Mux1/3
  Rotation (R313') from Perifocal to ECI/1(R313) -> R313'/1, Product1/1
  Cos1/1 -> Mux1/1
  Product1/1 -> [r_N], r_N/1, To Workspace1/1
  theta/1 -> Sin1/1, Cos1/1
  r/1 -> Product2/1
  Product2/1 -> Product1/2

== system Project26/Orbital Mechanics and Attitude Error /Rotation from Inertial to Body Frame ==
  note: $\vec{S_B} = q_{BN}'\otimes [\vec{S_N};0]\otimes q_{BN}$
  note: Quaternion Rotation (Double Tensor Product)
  S_N : Inport
  q_BN : Inport  Port=2
  Demux : Demux
  Mux : Mux  Inputs=3
  Quaternion multiplication 1 : Subsystem
  Quaternion multiplication 2 : Subsystem
  Transformation in Quaternion : Subsystem
  Transpose : Gain  Gain=[-1 -1 -1 1]
  S_B : Outport
  wires:
  S_N/1 -> Transformation in Quaternion/1(S_N)
  Mux/1 -> S_B/1
  Transpose/1 -> Quaternion multiplication 1/1(q_BN')
  q_BN/1 -> Quaternion multiplication 2/2(q_BN), Transpose/1
  Transformation in Quaternion/1(q(S_N)) -> Quaternion multiplication 1/2(q(S_N))
  Quaternion multiplication 2/1(q(S_B)) -> Demux/1
  Quaternion multiplication 1/1(q1) -> Quaternion multiplication 2/1(q1)
  Demux/1 -> Mux/1
  Demux/2 -> Mux/2
  Demux/3 -> Mux/3

== system Project26/Orbital Mechanics and Attitude Error /Sun Inertial Direction ==
  Clock : Clock
  Cos : Trigonometry  Operator=cos
  Gain : Gain  Gain=n_sun
  Gain1 : Gain  Gain=cos(epsilon)
  Gain2 : Gain  Gain=sin(epsilon)
  Gain3 : Gain  Gain=R_sun
  Mux : Mux  Inputs=3
  Sin : Trigonometry
  S_N : Outport
  wires:
  Clock/1 -> Gain/1
  Gain/1 -> Cos/1, Sin/1
  Sin/1 -> Gain2/1, Gain1/1
  Cos/1 -> Mux/1
  Gain1/1 -> Mux/2
  Gain2/1 -> Mux/3
  Mux/1 -> Gain3/1
  Gain3/1 -> S_N/1

== system Project26/Orbital Mechanics and Attitude Error /Theta angle ==
  note: Computation of theta angle from orbital parameters
      | a: Semi-major axis
      | e: Eccentricity
      | i: Inclination
      |
      | n: Average rotational rate of the orbit
  note: $\dot{\theta} = \frac{n(1+ecos\theta)^2}{(1-e^2)^{3/2}}$
  Constant : Constant
  Constant1 : Constant  Value=e
  Constant2 : Constant
  Constant3 : Constant  Value=3/2
  Constant4 : Constant  Value=theta0
  Cos : Trigonometry  Operator=cos
  Divide : Product  Inputs=*/
  Gain : Gain  Gain=e
  Gain1 : Gain  Gain=n
  Integrator : Integrator  InitialConditionSource=external
  Power : Math  Operator=pow
  Square : Math  Operator=square
  Square1 : Math  Operator=square
  Sum : Sum  Inputs=|++
  Sum1 : Sum  Inputs=|-+
  To Workspace : ToWorkspace  VariableName=theta  SampleTime=-1
  theta : Outport
  wires:
  Integrator/1 -> Cos/1, To Workspace/1, theta/1
  Cos/1 -> Gain/1
  Constant/1 -> Sum/1
  Gain/1 -> Sum/2
  Sum/1 -> Square/1
  Square/1 -> Gain1/1
  Constant1/1 -> Square1/1
  Square1/1 -> Sum1/1
  Constant2/1 -> Sum1/2
  Constant3/1 -> Power/2
  Sum1/1 -> Power/1
  Power/1 -> Divide/2
  Gain1/1 -> Divide/1
  Divide/1 -> Integrator/1
  Constant4/1 -> Integrator/2

== system Project26/Orbital Mechanics and Attitude Error /r (Magnitude) ==
  note: $r = \frac{a(1-e^2)}{1+ecos\theta}$
  note: Computation of radius r from orbital parameters
      | a: Semi-major axis
      | e: Eccentricity
      | i: Inclination
      |
      | n: Average rotational rate of the orbit
  theta : Inport
  Constant : Constant
  Constant1 : Constant  Value=e
  Constant2 : Constant
  Cos : Trigonometry  Operator=cos
  Divide : Product  Inputs=*/
  Gain : Gain  Gain=a
  Gain1 : Gain  Gain=e
  Square1 : Math  Operator=square
  Sum : Sum  Inputs=|++
  Sum1 : Sum  Inputs=|-+
  To Workspace : ToWorkspace  VariableName=rnorm  SampleTime=-1
  "r " : Outport
  wires:
  Constant1/1 -> Square1/1
  Square1/1 -> Sum1/1
  Constant2/1 -> Sum1/2
  Sum1/1 -> Gain/1
  theta/1 -> Cos/1
  Cos/1 -> Gain1/1
  Constant/1 -> Sum/1
  Gain1/1 -> Sum/2
  Gain/1 -> Divide/1
  Sum/1 -> Divide/2
  Divide/1 -> To Workspace/1, "r "/1

== system Project26/Sensors/Gyroscopes ==
  note: Angular Velocity
      | measured by Gyroscopes
  w_BN : Inport
  Band-Limited White Noise : simulink/Sources/Band-Limited White Noise  Cov=sensors.gyro.sigma_n^2*sensors.gyro.Ts  Ts=Tsample  seed=[23341]
  Band-Limited White Noise1 : simulink/Sources/Band-Limited White Noise  Cov=sensors.gyro.sigma_b^2*sensors.gyro.Ts  Ts=Tsample  seed=[23341]
  Integrator : Integrator  InitialCondition=sensors.gyro.RRW0
  Misalignment Error : Subsystem
  Resolution : Quantizer  QuantizationInterval=sensors.gyro.resolution
  Saturation (+/- 400°/s) : Saturate  UpperLimit=sensors.gyro.FS  LowerLimit=-sensors.gyro.FS
  Sum : Sum  Inputs=|+++
  To Workspace : ToWorkspace  VariableName=w_true  SampleTime=-1
  Zero-Order Hold : ZeroOrderHold  SampleTime=Tsample
  w_GYRO : Outport
  wires:
  w_BN/1 -> Misalignment Error/1(w_BN)
  Integrator/1 -> Sum/3
  Sum/1 -> Saturation (+/- 400°/s)/1
  Saturation (+/- 400°/s)/1 -> Resolution/1
  Resolution/1 -> Zero-Order Hold/1
  Zero-Order Hold/1 -> w_GYRO/1
  Band-Limited White Noise/1 -> Sum/2
  Band-Limited White Noise1/1 -> Integrator/1
  Misalignment Error/1(w (True Value)) -> To Workspace/1, Sum/1

== system Project26/Sensors/Magnetometer ==
  note: Magnetic Field
      | measured by Magnemeter
  note: Errors in the Measurements
  note: Magnetic Field
      | in Body Frame
      | (True value)
  B_B : Inport
  Gauss to Tesla Conversion : Gain  Gain=10^(-4)
  Hysteresis error : RandomNumber  Variance=((sensors.mag.hys/100*sensors.mag.FS/4)^2)*ones(3,1)  SampleTime=Tsample
  Linearity error : RandomNumber  Variance=((sensors.mag.lin/100*sensors.mag.FS/4)^2)*ones(3,1)  SampleTime=Tsample
  Non-Orthogonality Error : Subsystem
  Repeatibility error : RandomNumber  Variance=((sensors.mag.rep/100*sensors.mag.FS/4)^2)*ones(3,1)  SampleTime=Tsample
  "Resolution " : Quantizer  QuantizationInterval=sensors.mag.res
  Saturation Interval : Saturate  UpperLimit=sensors.mag.FS  LowerLimit=-sensors.mag.FS
  Sum1 : Sum  Inputs=|++++
  Tesla to Gauss Conversion : Gain  Gain=10^4
  To Workspace : ToWorkspace  VariableName=B_B_true  SampleTime=-1
  Zero-Order Hold1 : ZeroOrderHold  SampleTime=Tsample
  B_B_MM : Outport
  wires:
  Saturation Interval/1 -> "Resolution "/1
  B_B/1 -> Non-Orthogonality Error/1(B_B)
  Tesla to Gauss Conversion/1 -> Sum1/1
  Linearity error/1 -> Sum1/2
  Repeatibility error/1 -> Sum1/3
  Hysteresis error/1 -> Sum1/4
  Gauss to Tesla Conversion/1 -> B_B_MM/1
  Sum1/1 -> Saturation Interval/1
  "Resolution "/1 -> Zero-Order Hold1/1
  Zero-Order Hold1/1 -> Gauss to Tesla Conversion/1
  Non-Orthogonality Error/1(B_B (True)) -> Tesla to Gauss Conversion/1, To Workspace/1

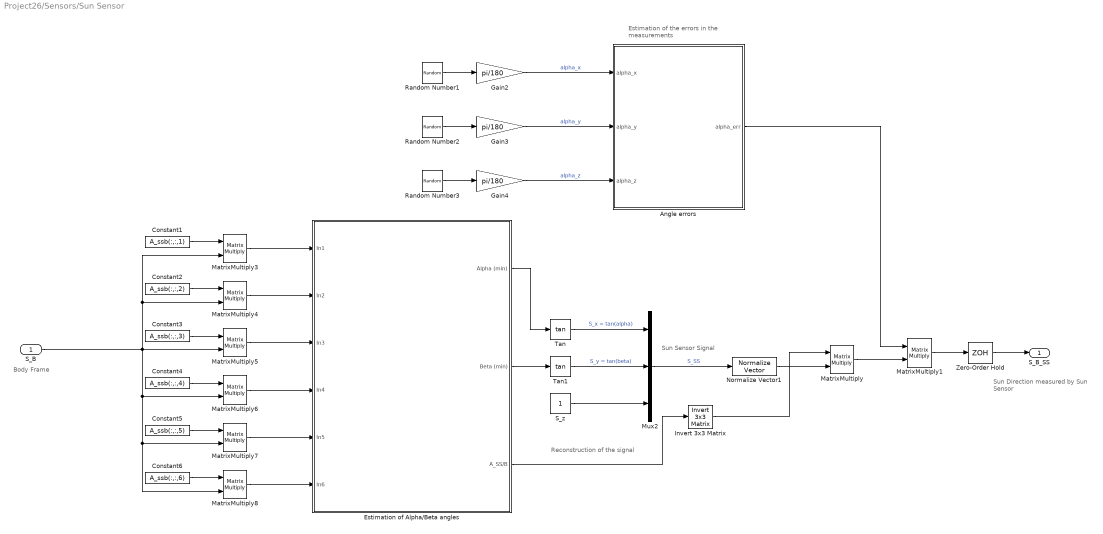
== system Project26/Sensors/Sun Sensor ==
  note: Sun Direction
      | measured by Sun Sensor
  note: Estimation of the
      | errors in the measurements
  note: Sun Sensor Signal
  note: Body Frame
  note: Reconstruction of the signal
  S_B : Inport
  Angle errors : Subsystem
  Constant1 : Constant  Value=A_ssb(:,:,1)  VectorParams1D=off
  Constant2 : Constant  Value=A_ssb(:,:,2)
  Constant3 : Constant  Value=A_ssb(:,:,3)
  Constant4 : Constant  Value=A_ssb(:,:,4)
  Constant5 : Constant  Value=A_ssb(:,:,5)
  Constant6 : Constant  Value=A_ssb(:,:,6)
  Estimation of Alpha/Beta angles : Subsystem
  Gain2 : Gain  Gain=pi/180
  Gain3 : Gain  Gain=pi/180
  Gain4 : Gain  Gain=pi/180
  Invert 3x3 Matrix : aerolibutil/Invert  3x3 Matrix
  MatrixMultiply{,1,3..8} (8 alike) : Product  Multiplication=Matrix(*)
  Mux2 : Mux  Inputs=3
  Normalize Vector1 : vrlib/Utilities/Normalize Vector  maxzero=0
  Random Number1 : RandomNumber  Variance=sensors.SS.accuracy^2  SampleTime=Tsample
  Random Number2 : RandomNumber  Variance=sensors.SS.accuracy^2  SampleTime=Tsample
  Random Number3 : RandomNumber  Variance=sensors.SS.accuracy^2  SampleTime=Tsample
  S_z : Constant
  Tan : Trigonometry  Operator=tan
  Tan1 : Trigonometry  Operator=tan
  Zero-Order Hold : ZeroOrderHold  SampleTime=Tsample
  S_B_SS : Outport
  wires:
  Estimation of Alpha/Beta angles/2(Beta (min)) -> Tan1/1
  Constant6/1 -> MatrixMultiply8/1
  Gain2/1 -> Angle errors/1(alpha_x)  "alpha_x"
  Invert 3x3 Matrix/1 -> MatrixMultiply/1
  Constant5/1 -> MatrixMultiply7/1
  MatrixMultiply4/1 -> Estimation of Alpha/Beta angles/2(In2)
  Constant3/1 -> MatrixMultiply5/1
  S_B/1 -> MatrixMultiply3/2, MatrixMultiply4/2, MatrixMultiply8/2, MatrixMultiply7/2, MatrixMultiply6/2, MatrixMultiply5/2
  MatrixMultiply1/1 -> Zero-Order Hold/1
  Constant1/1 -> MatrixMultiply3/1
  Constant2/1 -> MatrixMultiply4/1
  Mux2/1 -> Normalize Vector1/1  "S_SS"
  MatrixMultiply5/1 -> Estimation of Alpha/Beta angles/3(In3)
  Constant4/1 -> MatrixMultiply6/1
  Random Number3/1 -> Gain4/1
  MatrixMultiply/1 -> MatrixMultiply1/2
  Angle errors/1(alpha_err) -> MatrixMultiply1/1
  Tan/1 -> Mux2/1  "S_x = tan(alpha)"
  Random Number1/1 -> Gain2/1
  MatrixMultiply3/1 -> Estimation of Alpha/Beta angles/1(In1)
  S_z/1 -> Mux2/3
  Estimation of Alpha/Beta angles/1(Alpha (min)) -> Tan/1
  Gain3/1 -> Angle errors/2(alpha_y)  "alpha_y"
  Zero-Order Hold/1 -> S_B_SS/1
  Estimation of Alpha/Beta angles/3(A_SS/B) -> Invert 3x3 Matrix/1
  MatrixMultiply6/1 -> Estimation of Alpha/Beta angles/4(In4)
  Normalize Vector1/1 -> MatrixMultiply/2
  MatrixMultiply8/1 -> Estimation of Alpha/Beta angles/6(In6)
  Tan1/1 -> Mux2/2  "S_y = tan(beta)"
  MatrixMultiply7/1 -> Estimation of Alpha/Beta angles/5(In5)
  Random Number2/1 -> Gain3/1
  Gain4/1 -> Angle errors/3(alpha_z)  "alpha_z"

== system Project26/Attitude Determination/Enabled Subsystem/Kinematics ==
  note: Estimated
      | Quaternion
  w : Inport
  q_0 : Inport  Port=2
  Quaternion : Subsystem
      settings: PortSchema="{\"entries\":[{\"content\":{\"sides\":[{\"content\":{\"connectorIds\":[\"In1\"]},\"type\":\"ConnectorPlacement.EquallySpacedRectSide\",\"uuid\":\"337480c7-b996-434a-97d1-93b75d8b293c\"},{\"content\":{\"connectorIds\":[\"Out1\"],\"side\":\"RIGHT\"},\"type\":\"ConnectorPlacement.EquallySpacedRectSide\",\"uuid\":\"41d32615-4344-48a4-ad5b-2dad4deabdda\"},{\"content\":{\"side\":\"TOP\"},\"type\":\"ConnectorPlacement.EquallySpacedRectSide\",\"uuid\":\"47835596-097d-48d1-90ae-77b48fddf76d\"},{\"content\":{\"connectorIds\":[\"In2\",\"In3\"],\"side\":\"BOTTOM\"},\"type\":\"ConnectorPlacement.EquallySpacedRectSide\",\"uuid\":\"9f38fa4d-c6c1-4321-9750-02b4f73c744f\"}]},\"type\":\"ConnectorPlacement.EquallySpacedConnector\",\"uuid\":\"8ea16f6d-57f4-43cd-ae9c-44a64026dd8f\"}],\"packageUris\":[\"http://schema.mathworks.com/mf0/Connector/R2020b\"],\"version\":\"1.0\"}"
  Quaternion Normalization : Subsystem
  q_est : Outport
  wires:
  w/1 -> Quaternion/1(w)
  Quaternion Normalization/1(q_BN) -> Quaternion/3(q_BN), q_est/1  "q_BN = q normalized"
  Quaternion/1(q(t)) -> Quaternion Normalization/1(q(t))
  q_0/1 -> Quaternion/2(q_0)

== system Project26/Attitude Determination/Enabled Subsystem/Sign Determination ==
  "q_est " : Inport
  q_BN : Inport  Port=2
  Function to determinate the correct sign of the estimated quaternion : MATLAB Function  TreatAsAtomicUnit=on
  Subsystem : Subsystem
  q_est : Outport
  wires:
  Subsystem/1(Out1) -> q_est/1
  "q_est "/1 -> Function to determinate the correct sign of the estimated quaternion/2("q_est ")
  q_BN/1 -> Function to determinate the correct sign of the estimated quaternion/1(q_BN)
  Function to determinate the correct sign of the estimated quaternion/1(q_est) -> Subsystem/1(q_est)

== system Project26/Attitude Determination/Enabled Subsystem1/Sign determination ==
  "q_est " : Inport
  q_BN : Inport  Port=2
  Function to determinate the correct sign of the estimated quaternion : MATLAB Function  TreatAsAtomicUnit=on
  Subsystem : Subsystem
  To Workspace : ToWorkspace  VariableName=q_est1  SampleTime=-1
  q_0 : Outport
  wires:
  Subsystem/1(Out1) -> q_0/1
  "q_est "/1 -> To Workspace/1, Function to determinate the correct sign of the estimated quaternion/2("q_est ")
  q_BN/1 -> Function to determinate the correct sign of the estimated quaternion/1(q_BN)
  Function to determinate the correct sign of the estimated quaternion/1(q_est) -> Subsystem/1(q_est)

== system Project26/Control Logic/Control Block/Detumbling ==
  note: $\vec{M}_{detumbling} = - k_{d} \ (\vec{\omega} - \vec{\omega}_{d})$
  note: Proportional control
  note: Proportional coefficient of
      | Detumbling Controller
  w_obs : Inport
  q_obs : Inport  Port=2
  q_LN : Inport  Port=3
  Action Port : ActionPort  ActionPortLabel=if(u1<=u2)
  Constant : Constant  Value=control.detumbling.wd
  Gain : Gain  Gain=-control.detumbling.kd
  Pointing Error for Detumbling : Subsystem
  Rotation of w_DET : Subsystem
      settings: PortSchema="{\"entries\":[{\"content\":{\"sides\":[{\"content\":{\"connectorIds\":[\"In1\"]},\"type\":\"ConnectorPlacement.EquallySpacedRectSide\",\"uuid\":\"e766ba7c-a90d-4477-9792-9e015694ef4b\"},{\"content\":{\"side\":\"RIGHT\"},\"type\":\"ConnectorPlacement.EquallySpacedRectSide\",\"uuid\":\"09ef99fb-b530-4892-96c7-55e142825948\"},{\"content\":{\"connectorIds\":[\"Out1\"],\"side\":\"TOP\"},\"type\":\"ConnectorPlacement.EquallySpacedRectSide\",\"uuid\":\"c8b81143-c7b7-4fa7-b529-a6276f01a0c3\"},{\"content\":{\"connectorIds\":[\"In2\"],\"side\":\"BOTTOM\"},\"type\":\"ConnectorPlacement.EquallySpacedRectSide\",\"uuid\":\"76fccb77-3544-4711-8a34-4136377d4714\"}]},\"type\":\"ConnectorPlacement.EquallySpacedConnector\",\"uuid\":\"1bd14f97-bc0c-4b6f-aeff-af9c0bb68a55\"}],\"packageUris\":[\"http://schema.mathworks.com/mf0/Connector/R2020b\"],\"version\":\"1.0\"}"
  Sum : Sum  Inputs=|+-
  MC : Outport
  Pointing Error (DT) : Outport  Port=2
  wires:
  w_obs/1 -> Sum/1
  Sum/1 -> Gain/1  "w_e"
  q_obs/1 -> Pointing Error for Detumbling/1(q_obs)
  Pointing Error for Detumbling/1(Pointing Error) -> Pointing Error (DT)/1
  Gain/1 -> MC/1
  q_LN/1 -> Pointing Error for Detumbling/2(q_LN)
  Constant/1 -> Rotation of w_DET/1(w_DET)
  Rotation of w_DET/1(w_det_body) -> Sum/2
  Pointing Error for Detumbling/2(q_err) -> Rotation of w_DET/2(q_err)

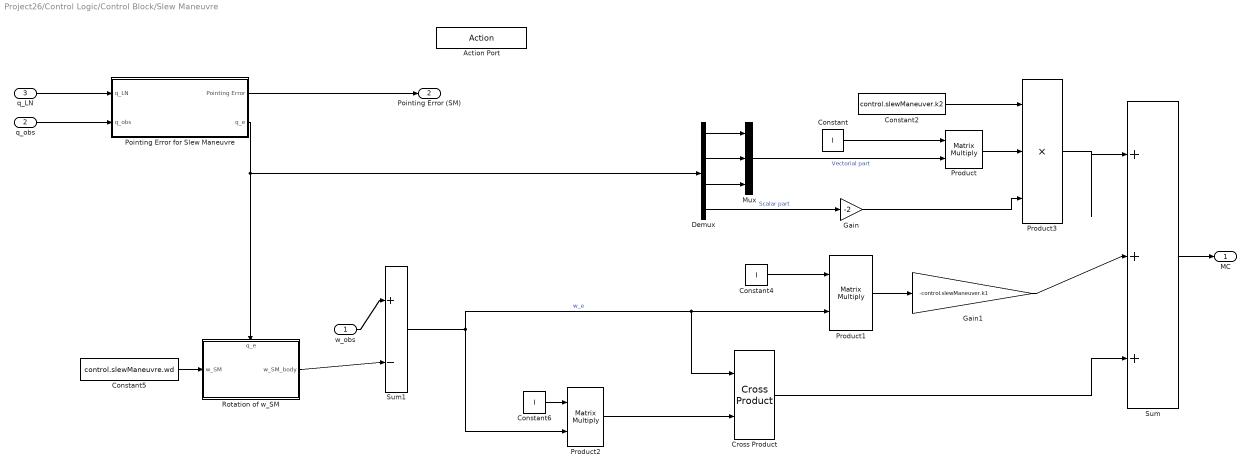
== system Project26/Control Logic/Control Block/Slew Maneuvre ==
  w_obs : Inport
  q_obs : Inport  Port=2
  q_LN : Inport  Port=3
  Action Port : ActionPort  ActionPortLabel=elseif(u2<u1<=u3)
  Constant : Constant  Value=I
  Constant2 : Constant  Value=control.slewManeuver.k2
  Constant4 : Constant  Value=I
  Constant5 : Constant  Value=control.slewManeuvre.wd
  Constant6 : Constant  Value=I
  Cross Product : matrix_library/Cross Product
  Demux : Demux
  Gain : Gain  Gain=-2
  Gain1 : Gain  Gain=-control.slewManeuver.k1
  Mux : Mux  Inputs=3
  Pointing Error for Slew Maneuvre : Subsystem
  Product : Product  Multiplication=Matrix(*)
  Product1 : Product  Multiplication=Matrix(*)
  Product2 : Product  Multiplication=Matrix(*)
  Product3 : Product  Inputs=3
  Rotation of w_SM : Subsystem
      settings: PortSchema="{\"entries\":[{\"content\":{\"sides\":[{\"content\":{\"connectorIds\":[\"In1\"]},\"type\":\"ConnectorPlacement.EquallySpacedRectSide\",\"uuid\":\"e766ba7c-a90d-4477-9792-9e015694ef4b\"},{\"content\":{\"connectorIds\":[\"Out1\"],\"side\":\"RIGHT\"},\"type\":\"ConnectorPlacement.EquallySpacedRectSide\",\"uuid\":\"09ef99fb-b530-4892-96c7-55e142825948\"},{\"content\":{\"connectorIds\":[\"In2\"],\"side\":\"TOP\"},\"type\":\"ConnectorPlacement.EquallySpacedRectSide\",\"uuid\":\"c8b81143-c7b7-4fa7-b529-a6276f01a0c3\"}]},\"type\":\"ConnectorPlacement.EquallySpacedConnector\",\"uuid\":\"1bd14f97-bc0c-4b6f-aeff-af9c0bb68a55\"}],\"packageUris\":[\"http://schema.mathworks.com/mf0/Connector/R2020b\"],\"version\":\"1.0\"}"
  Sum : Sum  Inputs=|+++
  Sum1 : Sum  Inputs=|+-
  MC : Outport
  Pointing Error (SM) : Outport  Port=2
  wires:
  Pointing Error for Slew Maneuvre/2(q_e) -> Rotation of w_SM/2(q_e), Demux/1
  Demux/3 -> Mux/3
  Demux/2 -> Mux/2
  Demux/1 -> Mux/1
  Demux/4 -> Gain/1  "Scalar part"
  Sum1/1 -> Product1/2, Cross Product/1, Product2/2  "w_e"
  Product2/1 -> Cross Product/2
  Constant6/1 -> Product2/1
  Cross Product/1 -> Sum/3
  Sum/1 -> MC/1
  Pointing Error for Slew Maneuvre/1(Pointing Error) -> Pointing Error (SM)/1
  Constant4/1 -> Product1/1
  Product1/1 -> Gain1/1
  Gain1/1 -> Sum/2
  Constant/1 -> Product/1
  Mux/1 -> Product/2  "Vectorial part"
  Constant2/1 -> Product3/1
  Product/1 -> Product3/2
  Gain/1 -> Product3/3
  Product3/1 -> Sum/1
  w_obs/1 -> Sum1/1
  q_LN/1 -> Pointing Error for Slew Maneuvre/1(q_LN)
  Constant5/1 -> Rotation of w_SM/1(w_SM)
  Rotation of w_SM/1(w_SM_body) -> Sum1/2
  q_obs/1 -> Pointing Error for Slew Maneuvre/2(q_obs)

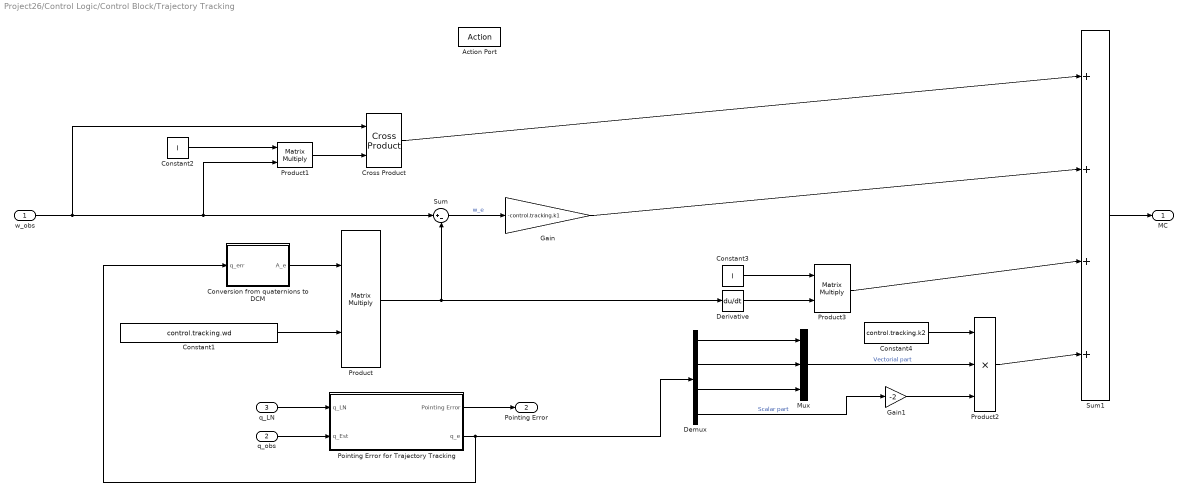
== system Project26/Control Logic/Control Block/Trajectory Tracking ==
  w_obs : Inport
  q_obs : Inport  Port=2
  q_LN : Inport  Port=3
  Action Port : ActionPort  ActionPortLabel=else
  Constant1 : Constant  Value=control.tracking.wd
  Constant2 : Constant  Value=I
  Constant3 : Constant  Value=I
  Constant4 : Constant  Value=control.tracking.k2
  Conversion from quaternions to DCM : Subsystem
  Cross Product : matrix_library/Cross Product
  Demux : Demux
  Derivative : Derivative
  Gain : Gain  Gain=-control.tracking.k1
  Gain1 : Gain  Gain=-2
  Mux : Mux  Inputs=3
  Pointing Error for Trajectory Tracking : Subsystem
  Product : Product  Multiplication=Matrix(*)
  Product1 : Product  Multiplication=Matrix(*)
  Product2 : Product  Inputs=3
  Product3 : Product  Multiplication=Matrix(*)
  Sum : Sum  Inputs=|+-
  Sum1 : Sum  Inputs=|++++
  MC : Outport
  Pointing Error : Outport  Port=2
  wires:
  q_obs/1 -> Pointing Error for Trajectory Tracking/2(q_Est)
  Conversion from quaternions to DCM/1(A_e) -> Product/1
  Product/1 -> Derivative/1, Sum/2
  Sum/1 -> Gain/1  "w_e"
  Product1/1 -> Cross Product/2
  Constant2/1 -> Product1/1
  Gain/1 -> Sum1/2
  Cross Product/1 -> Sum1/1
  Constant4/1 -> Product2/1
  Demux/1 -> Mux/1
  Demux/3 -> Mux/3
  Product2/1 -> Sum1/4
  Demux/2 -> Mux/2
  Demux/4 -> Gain1/1  "Scalar part"
  Product3/1 -> Sum1/3
  Constant3/1 -> Product3/1
  Derivative/1 -> Product3/2
  Sum1/1 -> MC/1
  Mux/1 -> Product2/2  "Vectorial part"
  Gain1/1 -> Product2/3
  w_obs/1 -> Sum/1, Product1/2, Cross Product/1
  q_LN/1 -> Pointing Error for Trajectory Tracking/1(q_LN)
  Constant1/1 -> Product/2
  Pointing Error for Trajectory Tracking/1(Pointing Error) -> Pointing Error/1
  Pointing Error for Trajectory Tracking/2(q_e) -> Conversion from quaternions to DCM/1(q_err), Demux/1

== system Project26/Control Logic/State Observer/OMEGA Matrix ==
  w_est_obs : Inport
  Demux : Demux  Outputs=3
  Gain1 : Gain  Gain=[0 0 0 1;0 0 1 0;0 -1 0 0;-1 0 0 0]
  Gain2 : Gain  Gain=[0 0 -1 0;0 0 0 1;1 0 0 0;0 -1 0 0]
  Gain3 : Gain  Gain=[0 1 0 0;-1 0 0 0;0 0 0 1;0 0 -1 0]
  Sum : Sum  Inputs=+++
  OMEGA : Outport
  wires:
  w_est_obs/1 -> Demux/1
  Sum/1 -> OMEGA/1
  Gain3/1 -> Sum/3
  Gain1/1 -> Sum/1
  Demux/2 -> Gain2/1
  Demux/1 -> Gain1/1
  Gain2/1 -> Sum/2
  Demux/3 -> Gain3/1

== system Project26/Control Logic/State Observer/Subsystem ==
  MC : Inport
  Demux : Demux  Outputs=3
  Mux : Mux  Inputs=3
  Out1 : Outport
  wires:
  MC/1 -> Demux/1
  Demux/1 -> Mux/1
  Demux/2 -> Mux/2
  Demux/3 -> Mux/3
  Mux/1 -> Out1/1

== system Project26/Disturbing Torques/Gravity Gradient Torque/Normalisation ==
  r_N : Inport
  Dot Product : DotProduct  OutDataTypeStr=Inherit: Inherit via internal rule
  Sqrt : Sqrt
  R : Outport
  wires:
  Dot Product/1 -> Sqrt/1
  r_N/1 -> Dot Product/1, Dot Product/2
  Sqrt/1 -> R/1

== system Project26/Disturbing Torques/Gravity Gradient Torque/Rotation of vector [1 0 0] ==
  note: Quaternion Rotation (Double Tensor Product)
  q_BL : Inport
  Vector [1 0 0] : Inport  Port=2
  Demux : Demux
  Mux : Mux  Inputs=3
  Quaternion multiplication 1 : Subsystem
  Quaternion multiplication 2 : Subsystem
  Transformation in Quaternion : Subsystem
  Transpose : Gain  Gain=[-1 -1 -1 1]
  v_rot : Outport
  wires:
  Vector [1 0 0]/1 -> Transformation in Quaternion/1(Vector [1 0 0])
  Mux/1 -> v_rot/1
  Transpose/1 -> Quaternion multiplication 1/1(q_BL)
  q_BL/1 -> Quaternion multiplication 2/2(q_BL), Transpose/1
  Transformation in Quaternion/1(q(vect)) -> Quaternion multiplication 1/2(q(vect))
  Quaternion multiplication 2/1(q(v_rot)) -> Demux/1
  Quaternion multiplication 1/1(q1) -> Quaternion multiplication 2/1(q1)
  Demux/1 -> Mux/1
  Demux/2 -> Mux/2
  Demux/3 -> Mux/3

== system Project26/Disturbing Torques/Magnetic Torque/Normalisation ==
  r_N : Inport
  Dot Product : DotProduct  OutDataTypeStr=Inherit: Inherit via internal rule
  Sqrt : Sqrt
  R : Outport
  wires:
  Dot Product/1 -> Sqrt/1
  r_N/1 -> Dot Product/1, Dot Product/2
  Sqrt/1 -> R/1
